simulink model "TNDProject"  (R2019b)
settings: Solver=VariableStepAuto  StartTime=0.0  StopTime=1.5  RelTol=1e-3
libraries: powerlib x50
settings Model: Creator=krish  LastModifiedBy=krish

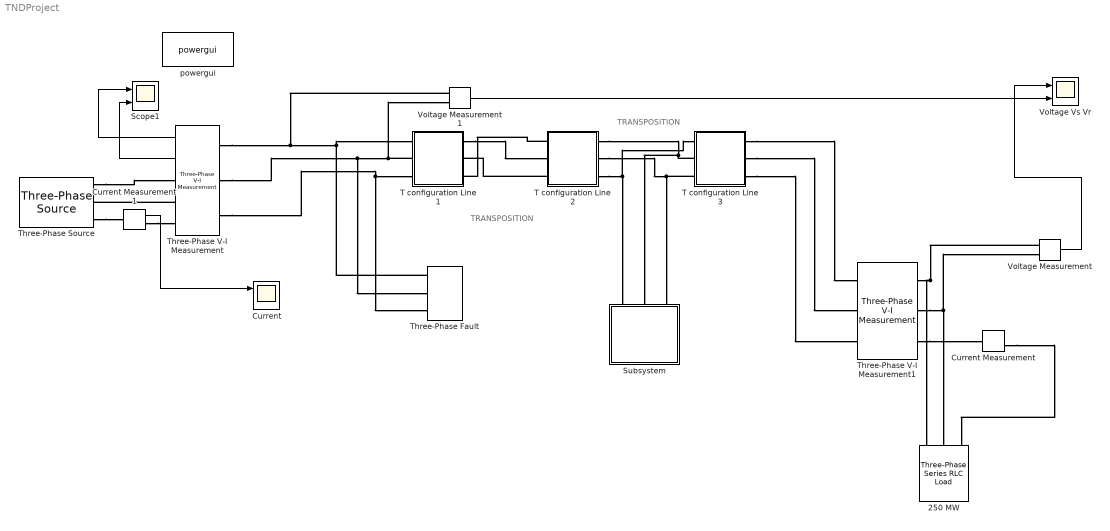
== system TNDProject ==
  note: TRANSPOSITION
  note: TRANSPOSITION
  250 MW : powerlib/Elements/Three-Phase Series RLC Load  LConnTagsString=A|B|C  Configuration=Y (grounded)  NominalVoltage=1000  Vabc=[1e3 1e3 1e3]  Vabcp=[1e3 1e3 1e3]  NominalFrequency=50  UnbalancedPower=off  ActivePower=10000  InductivePower=2500  CapacitivePower=500  Pabc=[10e3 9e3 11e3]  QLabc=[100 90 110]  QCabc=[100 90 110]  Pabcp=[10e3 9e3 11e3]  QLabcp=[100 90 110]  QCabcp=[100 90 110]  Measurements=None  LoadType=constant Z
      settings: SourceProductName=Simscape Electrical
  "Current " : Scope  NumInputPorts=2
  Current Measurement : powerlib/Measurements/Current Measurement  PhasorSimulation=off  OutputType=Complex  PSBequivalent=0
      settings: SourceProductName=Simscape Electrical
  Current Measurement1 : powerlib/Measurements/Current Measurement  PhasorSimulation=off  OutputType=Complex  PSBequivalent=0
      settings: SourceProductName=Simscape Electrical
  Scope1 : Scope  NumInputPorts=2
  Subsystem : Subsystem
      mask Display: fprintf("Compensation\nCapacitance")
  T configuration Line 1 : Subsystem
      mask Display:
      | %Line 1
      | fprintf("Line 1")
  T configuration Line 2 : Subsystem
      mask Display: fprintf("Line 2")
  T configuration Line 3 : Subsystem
      mask Display: fprintf("Line 3")
  Three-Phase V-I Measurement : powerlib/Measurements/Three-Phase V-I Measurement  VoltageMeasurement=phase-to-ground  SetLabelV=off  LabelV=Vabc  Vpu=off  VpuLL=off  CurrentMeasurement=yes  SetLabelI=off  LabelI=Iabc  Ipu=off  Pbase=100e6  Vbase=500e3  OutputType=Complex  PhasorSimulation=off  PSBequivalent=0
      settings: SourceProductName=Simscape Electrical
  Three-Phase V-I Measurement1 : powerlib/Measurements/Three-Phase V-I Measurement  VoltageMeasurement=phase-to-ground  SetLabelV=on  LabelV=Vabc  Vpu=off  VpuLL=off  CurrentMeasurement=yes  SetLabelI=on  LabelI=Iabc  Ipu=off  Pbase=100e6  Vbase=500e3  OutputType=Complex  PhasorSimulation=off  PSBequivalent=0
      settings: SourceProductName=Simscape Electrical
  "Three-Phase Fault " : powerlib/Elements/Three-Phase Fault  InitialStates=0  FaultA=on  FaultB=on  FaultC=on  GroundFault=on  SwitchTimes="[1/50  5/50]"  External=off  SwitchStatus=NaN  FaultResistance=0.001  GroundResistance=0.01  SnubberResistance=1e6  SnubberCapacitance=inf  Measurements=None
      settings: SourceProductName=Simscape Electrical
  Three-Phase Source : powerlib/Electrical Sources/Three-Phase Source  InternalConnection=Yg  VoltagePhases=off  Voltage=87e03  PhaseAngle=0  Voltage_phases=[25e3 25e3 25e3]/sqrt(3)  PhaseAngles_phases=[0 -120 +120]  Frequency=50  NonIdealSource=on  SpecifyImpedance=off  Resistance=0.8929  Inductance=16.58e-3  ShortCircuitLevel=100e6  BaseVoltage=25e3  XRratio=7  BusType=swing  Pref=10e3  Qref=0  Prefabc=[10e3, 10e3, 10e3]  Qrefabc=[0, 0, 0]  Qmin=-inf  Qmax=inf
      settings: SourceProductName=Simscape Electrical
  Voltage Measurement : powerlib/Measurements/Voltage Measurement  PhasorSimulation=off  OutputType=Complex  PSBequivalent=0
      settings: SourceProductName=Simscape Electrical
  Voltage Measurement1 : powerlib/Measurements/Voltage Measurement  PhasorSimulation=off  OutputType=Complex  PSBequivalent=0
      settings: SourceProductName=Simscape Electrical
  Voltage Vs Vr : Scope  NumInputPorts=2
  powergui : powerlib/powergui  Priority=1  SimulationMode=Continuous  SampleTime=50e-6  frequency=60  Iterations=50  frequencyindice=50  Pbase=100e6  ErrMax=1e-4  UnitsV=kV  UnitsW=MW  buscounter=0  FunctionMessages=off  echomessages=off  EnableUseOfTLC=off  CurrentSourceSwitches=off  DisableSnubberDevices=off  DisableRonSwitches=off  DisableVfSwitches=off  DisplayEquations=off  AutomaticDiscreteSolvers=off  SolverType=Tustin/Backward Euler (TBE)  Interpol=off  ExternalGateDelay=off  methode=off  Ts=100  x0status=blocks  SPID=on  SwTol=0  HookPort=off  NonlinearTolerance=1e-4  nMaxIteration=100  ContinueOnMaxIteration=off  RestoreLinks=warning  ResistiveCurrentMeasurement=off  Frange=[0:2:500]  Ylog=off  Xlog=on  ShowGrid=off  save=off  variable=ZData  structure=0  ZoomFFT=off  StartTime=0.0  cycles=1  DisplayStyle=1  fundamental=60  FreqAxis=off  MaxFrequency=1000  frequencyindicesteady=1  RmsSteady=1  display=off
      settings: SourceProductName=Simscape Electrical
  wires:
  Three-Phase V-I Measurement/2 -> Scope1/2
  Three-Phase V-I Measurement/1 -> Scope1/1
  Voltage Measurement/1 -> Voltage Vs Vr/1
  Current Measurement1/1 -> "Current "/1
  Voltage Measurement1/1 -> Voltage Vs Vr/2
  connections:
  Three-Phase Source/RConn1 -- Three-Phase V-I Measurement/RConn1
  Three-Phase V-I Measurement/RConn2 -- Three-Phase Source/RConn2
  Current Measurement1/RConn1 -- Three-Phase V-I Measurement/RConn3
  Three-Phase V-I Measurement/LConn1 -- Voltage Measurement1/LConn1 -- T configuration Line 1/LConn1 -- "Three-Phase Fault "/LConn1
  Three-Phase V-I Measurement1/RConn1 -- 250 MW/LConn1 -- Voltage Measurement/LConn1
  Three-Phase V-I Measurement1/RConn2 -- Voltage Measurement/LConn2 -- 250 MW/LConn2
  Current Measurement/RConn1 -- 250 MW/LConn3
  Three-Phase V-I Measurement1/RConn3 -- Current Measurement/LConn1
  T configuration Line 2/RConn1 -- T configuration Line 3/LConn2 -- Subsystem/LConn2
  T configuration Line 2/RConn2 -- T configuration Line 3/LConn3 -- Subsystem/LConn3
  T configuration Line 3/LConn1 -- Subsystem/LConn1 -- T configuration Line 2/RConn3
  Three-Phase Source/RConn3 -- Current Measurement1/LConn1
  Three-Phase V-I Measurement/LConn3 -- T configuration Line 1/LConn3 -- "Three-Phase Fault "/LConn3
  Three-Phase V-I Measurement/LConn2 -- T configuration Line 1/LConn2 -- Voltage Measurement1/LConn2 -- "Three-Phase Fault "/LConn2
  T configuration Line 2/LConn3 -- T configuration Line 1/RConn2
  T configuration Line 2/LConn1 -- T configuration Line 1/RConn3
  T configuration Line 1/RConn1 -- T configuration Line 2/LConn2
  T configuration Line 3/RConn1 -- Three-Phase V-I Measurement1/LConn1
  T configuration Line 3/RConn2 -- Three-Phase V-I Measurement1/LConn2
  T configuration Line 3/RConn3 -- Three-Phase V-I Measurement1/LConn3

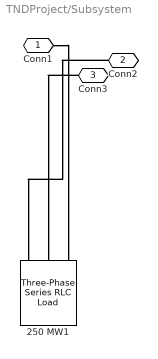
== system TNDProject/Subsystem ==
  250 MW1 : powerlib/Elements/Three-Phase Series RLC Load  LConnTagsString=A|B|C  Configuration=Y (grounded)  NominalVoltage=1000  Vabc=[1e3 1e3 1e3]  Vabcp=[1e3 1e3 1e3]  NominalFrequency=50  UnbalancedPower=off  ActivePower=2500  InductivePower=0  CapacitivePower=150  Pabc=[10e3 9e3 11e3]  QLabc=[100 90 110]  QCabc=[100 90 110]  Pabcp=[10e3 9e3 11e3]  QLabcp=[100 90 110]  QCabcp=[100 90 110]  Measurements=None  LoadType=constant Z
      settings: SourceProductName=Simscape Electrical
  Conn1 : PMIOPort  Side=Left
  Conn2 : PMIOPort  Port=2  Side=Left
  Conn3 : PMIOPort  Port=3  Side=Left
  connections:
  Conn2/RConn1 -- 250 MW1/LConn1
  Conn1/RConn1 -- 250 MW1/LConn3
  Conn3/RConn1 -- 250 MW1/LConn2

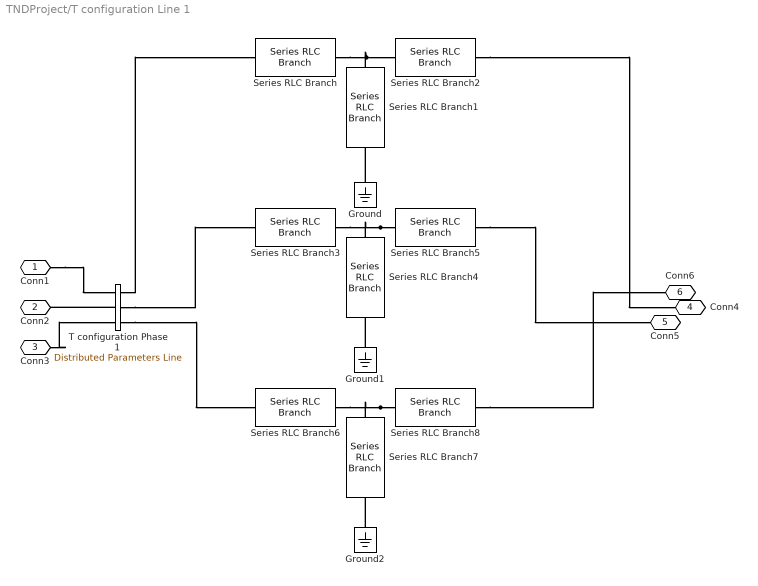
== system TNDProject/T configuration Line 1 ==
  Ground : powerlib/Elements/Ground  LConnTagsString=a
      settings: SourceProductName=Simscape Electrical
  Ground1 : powerlib/Elements/Ground  LConnTagsString=a
      settings: SourceProductName=Simscape Electrical
  Ground2 : powerlib/Elements/Ground  LConnTagsString=a
      settings: SourceProductName=Simscape Electrical
  Series RLC Branch{,2..3,5..6,8} (6 alike) : powerlib/Elements/Series RLC Branch  LConnTagsString=__new0  RConnTagsString=__new0  BranchType=RL  Resistance=1  Inductance=1e-3  SetiL0=off  InitialCurrent=0  Capacitance=1e-6  Setx0=off  InitialVoltage=0  Measurements=None
      settings: SourceProductName=Simscape Electrical
  Series RLC Branch1 : powerlib/Elements/Series RLC Branch  LConnTagsString=__new0  RConnTagsString=__new0  BranchType=C  Resistance=1  Inductance=1e-3  SetiL0=off  InitialCurrent=0  Capacitance=1e-6  Setx0=off  InitialVoltage=0  Measurements=None
      settings: SourceProductName=Simscape Electrical
  Series RLC Branch4 : powerlib/Elements/Series RLC Branch  LConnTagsString=__new0  RConnTagsString=__new0  BranchType=C  Resistance=1  Inductance=1e-3  SetiL0=off  InitialCurrent=0  Capacitance=1e-6  Setx0=off  InitialVoltage=0  Measurements=None
      settings: SourceProductName=Simscape Electrical
  Series RLC Branch7 : powerlib/Elements/Series RLC Branch  LConnTagsString=__new0  RConnTagsString=__new0  BranchType=C  Resistance=1  Inductance=1e-3  SetiL0=off  InitialCurrent=0  Capacitance=1e-6  Setx0=off  InitialVoltage=0  Measurements=None
      settings: SourceProductName=Simscape Electrical
  T configuration Phase 1 : powerlib/Elements/Distributed Parameters Line  Phases=3  Frequency=60  Resistance=[0.01273 0.3864]  Inductance="[0.9337e-3  4.1264e-3]"  Capacitance=[12.74e-9 7.751e-9]  Length=100  x1=[3.10829045531774e-11 74754.5317447537 74754.5317447536;314.159265358979 314.159265358979 314.159265358979;-2.96049210653657 0.387635773894008 -1.18316055290089]  x2=[1.99790959853941e-10 64973.0709424805 64973.0709424804;314.159265358979 314.159265358979 314.159265358979;-3.13615195954466 0.182704018298384 -1.38809230849651]  x3=[1.16687445957054e-12 393.930828866331 393.930828866331;314.159265358979 314.159265358979 314.159265358979;1.98441826894467 2.46456979807396 0.89377347127906]  x4=[1.67566370222132e-12 814.762514451291 814.76251445129;314.159265358979 314.159265358979 314.159265358979;-1.35875787866938 -0.155175511306906 -1.72597183810181]  x5=0.000565541566995742  V1=[3.108e-11 7.475e+04 7.475e+04;314.2 314.2 314.2;-2.96 0.3876 -1.183]  V2=[1.998e-10 6.497e+04 6.497e+04;314.2 314.2 314.2;-3.136 0.1827 -1.388]  I1=[1.167e-12 393.9 393.9;314.2 314.2 314.2;1.984 2.465 0.8938]  I2=[1.676e-12 814.8 814.8;314.2 314.2 314.2;-1.359 -0.1552 -1.726]  nHarmo=1  Measurements=None
      settings: SourceProductName=Simscape Electrical
  Conn1 : PMIOPort  Side=Left
  Conn2 : PMIOPort  Port=2  Side=Left
  Conn3 : PMIOPort  Port=3  Side=Left
  Conn4 : PMIOPort  Port=4  Side=Right
  Conn5 : PMIOPort  Port=5  Side=Right
  Conn6 : PMIOPort  Port=6  Side=Right
  connections:
  T configuration Phase 1/LConn2 -- Conn2/RConn1
  Series RLC Branch/RConn1 -- Series RLC Branch1/LConn1 -- Series RLC Branch2/LConn1
  Conn1/RConn1 -- T configuration Phase 1/LConn1
  Conn3/RConn1 -- T configuration Phase 1/LConn3
  T configuration Phase 1/RConn1 -- Series RLC Branch/LConn1
  Series RLC Branch2/RConn1 -- Conn4/RConn1
  Ground/LConn1 -- Series RLC Branch1/RConn1
  Series RLC Branch5/LConn1 -- Series RLC Branch3/RConn1 -- Series RLC Branch4/LConn1
  T configuration Phase 1/RConn2 -- Series RLC Branch3/LConn1
  Ground1/LConn1 -- Series RLC Branch4/RConn1
  Series RLC Branch5/RConn1 -- Conn5/RConn1
  Series RLC Branch8/LConn1 -- Series RLC Branch6/RConn1 -- Series RLC Branch7/LConn1
  T configuration Phase 1/RConn3 -- Series RLC Branch6/LConn1
  Ground2/LConn1 -- Series RLC Branch7/RConn1
  Series RLC Branch8/RConn1 -- Conn6/RConn1

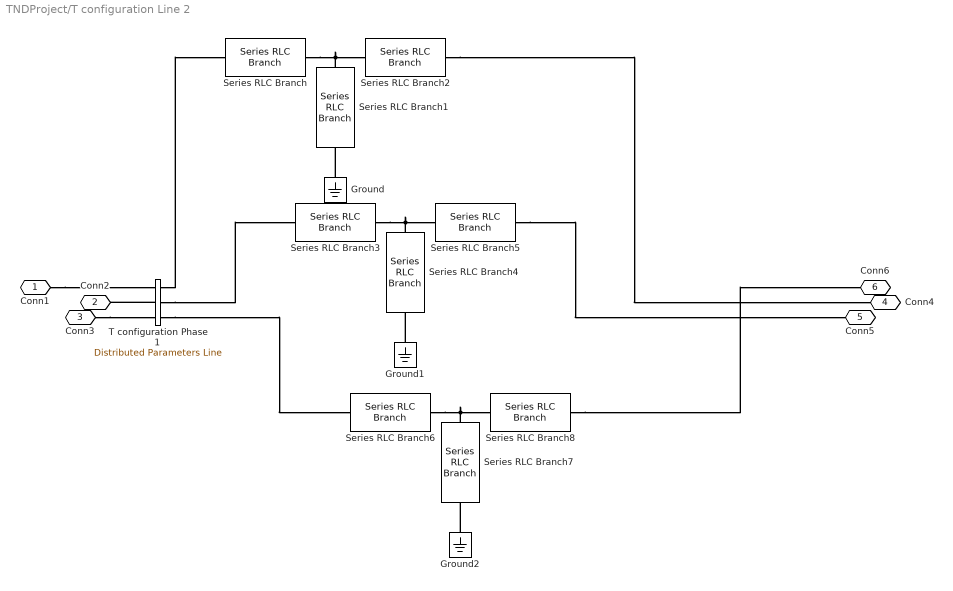
== system TNDProject/T configuration Line 2 ==
  Ground : powerlib/Elements/Ground  LConnTagsString=a
      settings: SourceProductName=Simscape Electrical
  Ground1 : powerlib/Elements/Ground  LConnTagsString=a
      settings: SourceProductName=Simscape Electrical
  Ground2 : powerlib/Elements/Ground  LConnTagsString=a
      settings: SourceProductName=Simscape Electrical
  Series RLC Branch{,2..3,5..6,8} (6 alike) : powerlib/Elements/Series RLC Branch  LConnTagsString=__new0  RConnTagsString=__new0  BranchType=RL  Resistance=1  Inductance=1e-3  SetiL0=off  InitialCurrent=0  Capacitance=1e-6  Setx0=off  InitialVoltage=0  Measurements=None
      settings: SourceProductName=Simscape Electrical
  Series RLC Branch1 : powerlib/Elements/Series RLC Branch  LConnTagsString=__new0  RConnTagsString=__new0  BranchType=C  Resistance=1  Inductance=1e-3  SetiL0=off  InitialCurrent=0  Capacitance=1e-6  Setx0=off  InitialVoltage=0  Measurements=None
      settings: SourceProductName=Simscape Electrical
  Series RLC Branch4 : powerlib/Elements/Series RLC Branch  LConnTagsString=__new0  RConnTagsString=__new0  BranchType=C  Resistance=1  Inductance=1e-3  SetiL0=off  InitialCurrent=0  Capacitance=1e-6  Setx0=off  InitialVoltage=0  Measurements=None
      settings: SourceProductName=Simscape Electrical
  Series RLC Branch7 : powerlib/Elements/Series RLC Branch  LConnTagsString=__new0  RConnTagsString=__new0  BranchType=C  Resistance=1  Inductance=1e-3  SetiL0=off  InitialCurrent=0  Capacitance=1e-6  Setx0=off  InitialVoltage=0  Measurements=None
      settings: SourceProductName=Simscape Electrical
  T configuration Phase 1 : powerlib/Elements/Distributed Parameters Line  Phases=3  Frequency=60  Resistance=[0.01273 0.3864]  Inductance="[0.9337e-3  4.1264e-3]"  Capacitance=[12.74e-9 7.751e-9]  Length=100  x1=[1.91987416502652e-10 63735.4267827208 63735.4267827208;314.159265358979 314.159265358979 314.159265358979;3.13530165676195 2.28067868153745 0.709882354742551]  x2=[1.76741756957581e-10 56190.3355636402 56190.3355636403;314.159265358979 314.159265358979 314.159265358979;3.11891927229639 2.00819499419854 0.43739866740364]  x3=[2.49206789016568e-13 414.419878777158 414.419878777155;314.159265358979 314.159265358979 314.159265358979;2.93615189377902 -1.64327618154293 3.06911279884176]  x4=[5.1037492748281e-13 814.312753280553 814.312753280552;314.159265358979 314.159265358979 314.159265358979;2.25529625824477 1.80713313074532 0.236336803950426]  x5=0.000565541566995742  V1=[1.92e-10 6.374e+04 6.374e+04;314.2 314.2 314.2;3.135 2.281 0.7099]  V2=[1.767e-10 5.619e+04 5.619e+04;314.2 314.2 314.2;3.119 2.008 0.4374]  I1=[2.492e-13 414.4 414.4;314.2 314.2 314.2;2.936 -1.643 3.069]  I2=[5.104e-13 814.3 814.3;314.2 314.2 314.2;2.255 1.807 0.2363]  nHarmo=1  Measurements=None
      settings: SourceProductName=Simscape Electrical
  Conn1 : PMIOPort  Side=Left
  Conn2 : PMIOPort  Port=2  Side=Left
  Conn3 : PMIOPort  Port=3  Side=Left
  Conn4 : PMIOPort  Port=4  Side=Right
  Conn5 : PMIOPort  Port=5  Side=Right
  Conn6 : PMIOPort  Port=6  Side=Right
  connections:
  T configuration Phase 1/LConn2 -- Conn2/RConn1
  Series RLC Branch/RConn1 -- Series RLC Branch2/LConn1 -- Series RLC Branch1/LConn1
  Conn1/RConn1 -- T configuration Phase 1/LConn1
  Conn3/RConn1 -- T configuration Phase 1/LConn3
  T configuration Phase 1/RConn1 -- Series RLC Branch/LConn1
  Series RLC Branch2/RConn1 -- Conn4/RConn1
  Ground/LConn1 -- Series RLC Branch1/RConn1
  Series RLC Branch4/LConn1 -- Series RLC Branch5/LConn1 -- Series RLC Branch3/RConn1
  T configuration Phase 1/RConn2 -- Series RLC Branch3/LConn1
  Ground1/LConn1 -- Series RLC Branch4/RConn1
  Series RLC Branch5/RConn1 -- Conn5/RConn1
  Series RLC Branch7/LConn1 -- Series RLC Branch8/LConn1 -- Series RLC Branch6/RConn1
  T configuration Phase 1/RConn3 -- Series RLC Branch6/LConn1
  Ground2/LConn1 -- Series RLC Branch7/RConn1
  Series RLC Branch8/RConn1 -- Conn6/RConn1

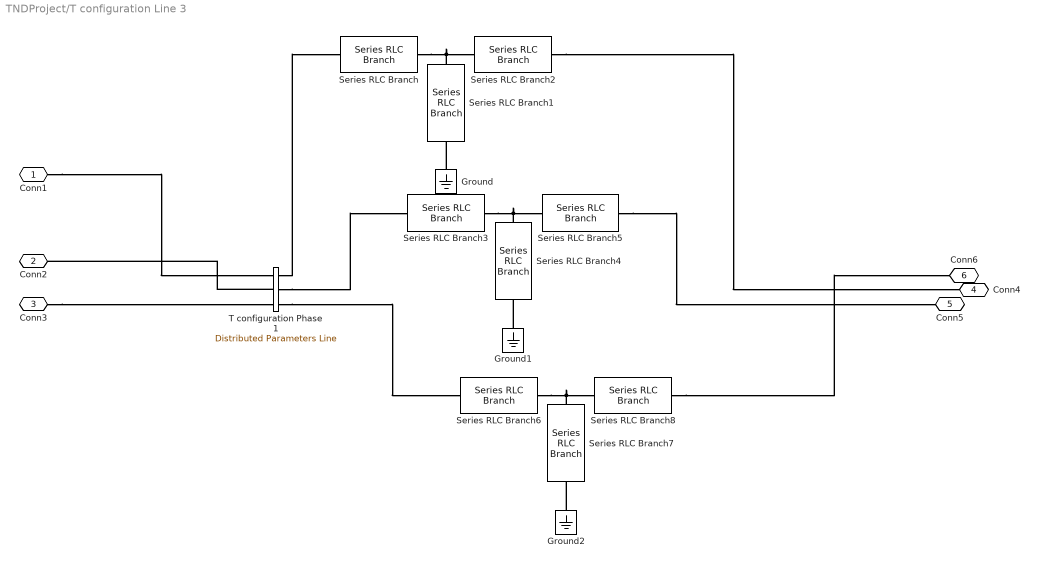
== system TNDProject/T configuration Line 3 ==
  Ground : powerlib/Elements/Ground  LConnTagsString=a
      settings: SourceProductName=Simscape Electrical
  Ground1 : powerlib/Elements/Ground  LConnTagsString=a
      settings: SourceProductName=Simscape Electrical
  Ground2 : powerlib/Elements/Ground  LConnTagsString=a
      settings: SourceProductName=Simscape Electrical
  Series RLC Branch{,2..3,5..6,8} (6 alike) : powerlib/Elements/Series RLC Branch  LConnTagsString=__new0  RConnTagsString=__new0  BranchType=RL  Resistance=1  Inductance=1e-3  SetiL0=off  InitialCurrent=0  Capacitance=1e-6  Setx0=off  InitialVoltage=0  Measurements=None
      settings: SourceProductName=Simscape Electrical
  Series RLC Branch1 : powerlib/Elements/Series RLC Branch  LConnTagsString=__new0  RConnTagsString=__new0  BranchType=C  Resistance=1  Inductance=1e-3  SetiL0=off  InitialCurrent=0  Capacitance=1e-6  Setx0=off  InitialVoltage=0  Measurements=None
      settings: SourceProductName=Simscape Electrical
  Series RLC Branch4 : powerlib/Elements/Series RLC Branch  LConnTagsString=__new0  RConnTagsString=__new0  BranchType=C  Resistance=1  Inductance=1e-3  SetiL0=off  InitialCurrent=0  Capacitance=1e-6  Setx0=off  InitialVoltage=0  Measurements=None
      settings: SourceProductName=Simscape Electrical
  Series RLC Branch7 : powerlib/Elements/Series RLC Branch  LConnTagsString=__new0  RConnTagsString=__new0  BranchType=C  Resistance=1  Inductance=1e-3  SetiL0=off  InitialCurrent=0  Capacitance=1e-6  Setx0=off  InitialVoltage=0  Measurements=None
      settings: SourceProductName=Simscape Electrical
  T configuration Phase 1 : powerlib/Elements/Distributed Parameters Line  Phases=3  Frequency=60  Resistance=[0.01273 0.3864]  Inductance="[0.9337e-3  4.1264e-3]"  Capacitance=[12.74e-9 7.751e-9]  Length=100  x1=[1.39635022496442e-10 54897.5047253939 54897.5047253939;314.159265358979 314.159265358979 314.159265358979;-3.08257776237914 -2.18111963106237 2.53126934932232]  x2=[8.375256171873e-11 50216.0265970974 50216.0265970975;314.159265358979 314.159265358979 314.159265358979;2.92047163498091 -2.44457114234126 2.26781783804343]  x3=[3.09460255099791e-13 314.506074389084 314.506074389083;314.159265358979 314.159265358979 314.159265358979;-1.28481884101144 0.319999049555291 -1.2507972772396]  x4=[9.44741156726808e-13 680.388334286176 680.388334286176;314.159265358979 314.159265358979 314.159265358979;2.4084287951069 -2.56803871306054 2.14435026732415]  x5=0.000565541566995742  V1=[1.396e-10 5.49e+04 5.49e+04;314.2 314.2 314.2;-3.083 -2.181 2.531]  V2=[8.375e-11 5.022e+04 5.022e+04;314.2 314.2 314.2;2.92 -2.445 2.268]  I1=[3.095e-13 314.5 314.5;314.2 314.2 314.2;-1.285 0.32 -1.251]  I2=[9.447e-13 680.4 680.4;314.2 314.2 314.2;2.408 -2.568 2.144]  nHarmo=1  Measurements=None
      settings: SourceProductName=Simscape Electrical
  Conn1 : PMIOPort  Side=Left
  Conn2 : PMIOPort  Port=2  Side=Left
  Conn3 : PMIOPort  Port=3  Side=Left
  Conn4 : PMIOPort  Port=4  Side=Right
  Conn5 : PMIOPort  Port=5  Side=Right
  Conn6 : PMIOPort  Port=6  Side=Right
  connections:
  T configuration Phase 1/LConn2 -- Conn2/RConn1
  Series RLC Branch/RConn1 -- Series RLC Branch2/LConn1 -- Series RLC Branch1/LConn1
  Conn1/RConn1 -- T configuration Phase 1/LConn1
  Conn3/RConn1 -- T configuration Phase 1/LConn3
  T configuration Phase 1/RConn1 -- Series RLC Branch/LConn1
  Series RLC Branch2/RConn1 -- Conn4/RConn1
  Ground/LConn1 -- Series RLC Branch1/RConn1
  Series RLC Branch4/LConn1 -- Series RLC Branch5/LConn1 -- Series RLC Branch3/RConn1
  T configuration Phase 1/RConn2 -- Series RLC Branch3/LConn1
  Ground1/LConn1 -- Series RLC Branch4/RConn1
  Series RLC Branch5/RConn1 -- Conn5/RConn1
  Series RLC Branch7/LConn1 -- Series RLC Branch8/LConn1 -- Series RLC Branch6/RConn1
  T configuration Phase 1/RConn3 -- Series RLC Branch6/LConn1
  Ground2/LConn1 -- Series RLC Branch7/RConn1
  Series RLC Branch8/RConn1 -- Conn6/RConn1
